simulink model "FOPDT"  (R2018b)
settings: Solver=FixedStepDiscrete  StartTime=0.0  StopTime=1800  FixedStep=1  RelTol=1e-3
settings Model: Creator=Trips  LastModifiedBy=Trips
settings ConfigComp: PLC_TargetIDE=step7  PLC_GenerateReport=off  PLC_LaunchReport=off

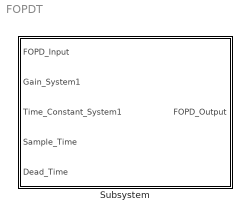
== system FOPDT ==
  Subsystem : Subsystem  TreatAsAtomicUnit=on

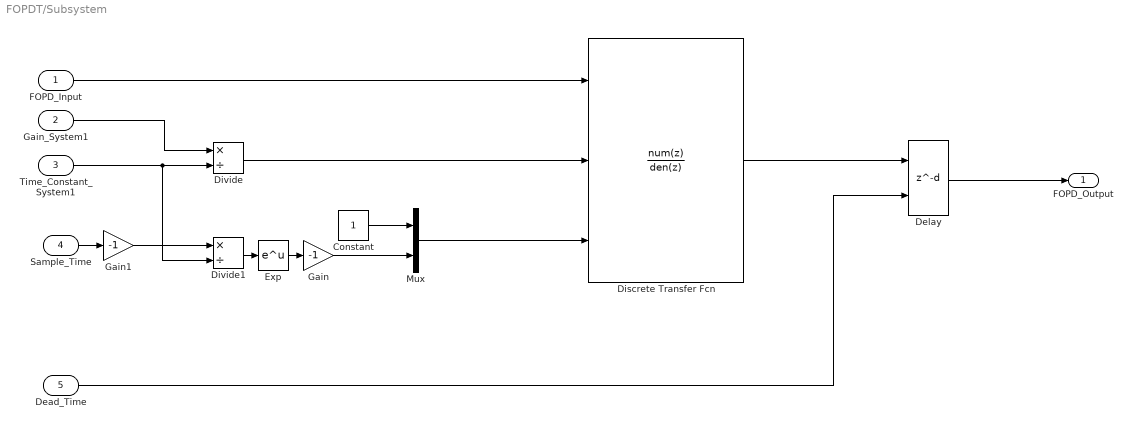
== system FOPDT/Subsystem ==
  FOPD_Input : Inport
  Gain_System1 : Inport  Port=2
  Time_Constant_System1 : Inport  Port=3
  Sample_Time : Inport  Port=4
  " Dead_Time" : Inport  Port=5
  Constant : Constant
  Delay : Delay  DelayLengthSource=Input port  DelayLength=600  DelayLengthUpperLimit=800
      settings: InputPortMap=u0,p1
  Discrete Transfer Fcn : DiscreteTransferFcn  NumeratorSource=Input port  DenominatorSource=Input port  a0EqualsOne=on
      settings: InputPortMap=u0,p1,p3
  Divide : Product  Inputs=*/
  Divide1 : Product  Inputs=*/
  Exp : Math  SaturateOnIntegerOverflow=on
  Gain : Gain  Gain=-1
  Gain1 : Gain  Gain=-1
  Mux : Mux  Inputs=2
  FOPD_Output : Outport
  wires:
  Gain1/1 -> Divide1/1
  Time_Constant_System1/1 -> Divide1/2, Divide/2
  FOPD_Input/1 -> Discrete Transfer Fcn/1
  Delay/1 -> FOPD_Output/1
  Divide/1 -> Discrete Transfer Fcn/2
  Exp/1 -> Gain/1
  Constant/1 -> Mux/1
  Mux/1 -> Discrete Transfer Fcn/3
  Divide1/1 -> Exp/1
  Discrete Transfer Fcn/1 -> Delay/1
  Gain_System1/1 -> Divide/1
  Gain/1 -> Mux/2
  " Dead_Time"/1 -> Delay/2
  Sample_Time/1 -> Gain1/1
